simulink model "CnvSet_Trq2Q"  (R2018a)
settings: configuration reference "cs_ert" (kept outside this file)
values from neighbouring files (symbols this model uses):
  PhyMod_trq2qBas_MAP = 0.0 6.3 12.7 17.5 24.7 31.5 37.5 46.1 57.2 63.06 71.16 79.26 87.36 95.46 103.56 111.66 0.0 5.8 12.1 16.76 23.5 30.46 36.7 45.0 53.36 62.06 70.16 78.26 86.36 94.46 102.56 110.66 0.0 5.4 11.5 16.0 22.3 29.4 36.3 43.6 52.6 61.3 69.4 77.5 85.6 93.7 101.8 109.9 0.0 5.6 12.0 16.6 20.5 27.4 34.9 40.8 47.6 54.5 60.8 67.3 74.8 82.8 89.8 97.8 0.0 5.8 12.1 16.8 20.9 26.6 34.6 40.46 46.96 53.7 60.3 67.1 74.16    [CnvSet_Trq2Q.sldd]
  PhyMod_trq2qBas_MAPX : value not decoded    [CnvSet_Trq2Q.sldd]
  PhyMod_trq2qBas_MAPY : value not decoded    [CnvSet_Trq2Q.sldd]
settings Model: DataDictionary=CnvSet_Trq2Q.sldd  Creator=zhoutinglin  LastModifiedBy=zhoutinglin

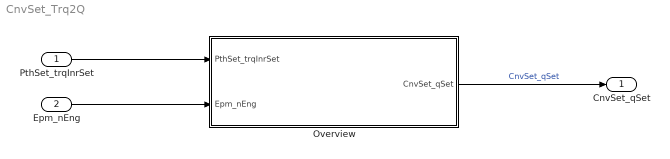
== system CnvSet_Trq2Q ==
  PthSet_trqInrSet : Inport  Description=Inner torque set value after monitoring limitation  OutMin=-3000  OutMax=3276.7  OutDataTypeStr=Torq  Unit=Nm  PortDimensions=[1 1]
  Epm_nEng : Inport  Description=Engine speed  Port=2  OutMin=0  OutMax=6000  OutDataTypeStr=ERPM  Unit=rpm  PortDimensions=[1 1]
  Overview : Subsystem
  CnvSet_qSet : Outport
  wires:
  PthSet_trqInrSet/1 -> Overview/1(PthSet_trqInrSet)
  Epm_nEng/1 -> Overview/2(Epm_nEng)
  Overview/1(CnvSet_qSet) -> CnvSet_qSet/1  "CnvSet_qSet"

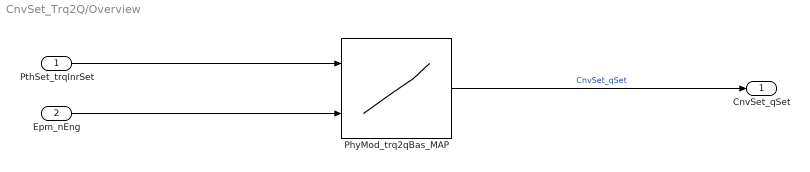
== system CnvSet_Trq2Q/Overview ==
  PthSet_trqInrSet : Inport  Tag=Nm
  Epm_nEng : Inport  Tag=rpm  Port=2
  PhyMod_trq2qBas_MAP : Lookup_n-D  BreakpointsForDimension1=PhyMod_trq2qBas_MAPY  BreakpointsForDimension2=PhyMod_trq2qBas_MAPX  BreakpointsForDimension1DataTypeStr=Inherit: Inherit from 'Breakpoint data'  BreakpointsForDimension2DataTypeStr=Inherit: Inherit from 'Breakpoint data'  Table=PhyMod_trq2qBas_MAP  TableDataTypeStr=Inherit: Inherit from 'Table data'  ExtrapMethod=Clip  InternalRulePriority=Speed  OutDataTypeStr=Inherit: Inherit from 'Table data'  RndMeth=Simplest
  CnvSet_qSet : Outport  Tag=mg/hub
  wires:
  PhyMod_trq2qBas_MAP/1 -> CnvSet_qSet/1  "CnvSet_qSet"
  Epm_nEng/1 -> PhyMod_trq2qBas_MAP/2
  PthSet_trqInrSet/1 -> PhyMod_trq2qBas_MAP/1
